simulink model "TPINVT"  (R2024b)
settings: Solver=VariableStepAuto  StartTime=0.0  StopTime=0.5  RelTol=1e-3
libraries: spsSeriesRLCBranchLib x6, spsVoltageMeasurementLib x3, spsCurrentMeasurementLib x2, spsDCVoltageSourceLib x1, simulink x1, spsUniversalBridgeLib x1, sps_lib x1
settings Model: Creator=李康诚  LastModifiedBy=86195
settings SolverCC: AlgebraicLoopSolver=TrustRegion
settings DebuggingCC: UnconnectedInputMsg=warning  UnconnectedOutputMsg=warning  UnconnectedLineMsg=warning
settings ModelReferenceCC: EnableRefExpFcnMdlSchedulingChecks=on
settings RTWCC: GPUComputeCapability=3.5  DLArmComputeVersion=19.05

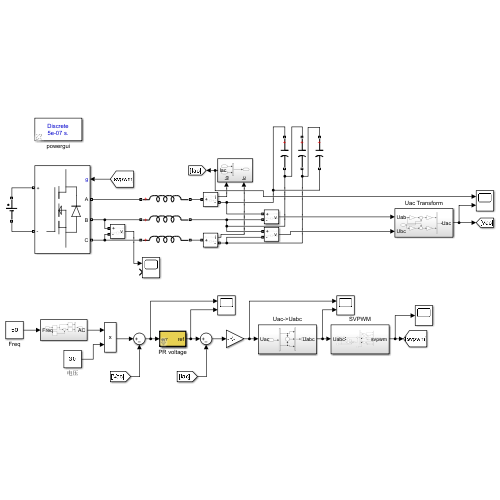
[thumbnail: Simulink's stored preview of the top-level diagram]
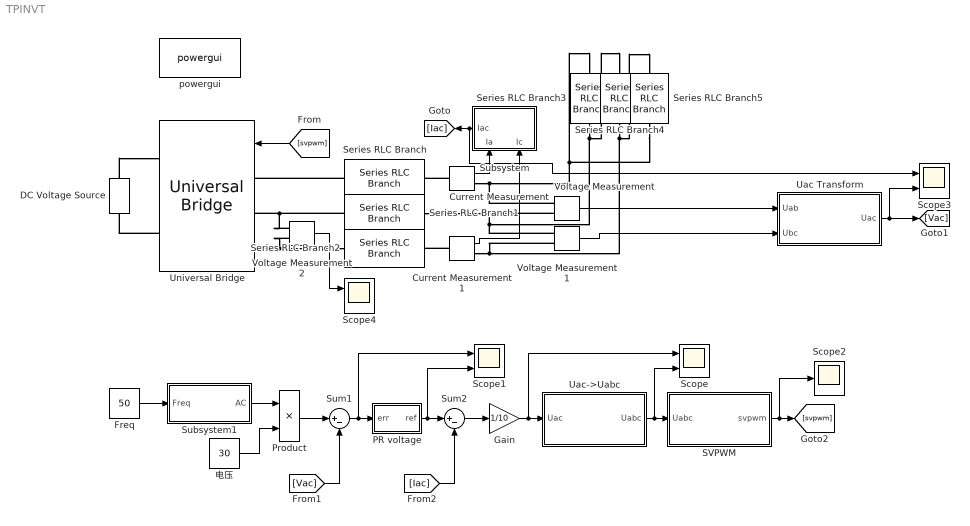
== system TPINVT ==
  Current Measurement : spsCurrentMeasurementLib/Current Measurement  PhasorSimulation=off  OutputType=Complex  PSBequivalent=0
  Current Measurement1 : spsCurrentMeasurementLib/Current Measurement  PhasorSimulation=off  OutputType=Complex  PSBequivalent=0
  DC Voltage Source : spsDCVoltageSourceLib/DC Voltage Source  Amplitude=50  Measurements=None
  Freq : Constant  Value=50
  Gain : Gain  Gain=1/10
  PR voltage : Subsystem  TreatAsAtomicUnit=on  mask{Kp=0.2, Kr=40, Wc=5, Upper=40, Lower=-40}
  Product : Product
  SVPWM : Subsystem
      settings: PortSchema="{\"entries\":[{\"content\":{\"sides\":[{\"content\":{\"connectorIds\":[\"Out1\"]},\"type\":\"ConnectorPlacement.EquallySpacedRectSide\",\"uuid\":\"dcbf9248-7910-4260-a5d4-f1c1a6bfbbe0\"},{\"content\":{\"connectorIds\":[\"In1\"],\"side\":\"RIGHT\"},\"type\":\"ConnectorPlacement.EquallySpacedRectSide\",\"uuid\":\"1c1c0724-ccc5-4c64-9077-43c2945212ef\"},{\"content\":{\"connectorIds\":[],\"side\":\"TOP\"},\"type\":\"ConnectorPlacement.EquallySpacedRectSide\",\"uuid\":\"9c7778fd-5bd1-45c2-a026-753aafe02b02\"},{\"content\":{\"connectorIds\":[],\"side\":\"HIDDEN\"},\"type\":\"ConnectorPlacement.EquallySpacedRectSide\",\"uuid\":\"bbcc7e5f-60a4-4189-91e6-d18a042c4fa5\"}]},\"type\":\"ConnectorPlacement.EquallySpacedConnector\",\"uuid\":\"5934fde8-9463-4fa5-a9de-717ebb1e8e0c\"}],\"packageUris\":[\"http://schema.mathworks.com/mf0/Connector/R2020b\"],\"version\":\"1.0\"}"
  Scope{,1,3..4} (4 alike) : Scope  NumInputPorts=2
  Scope2 : Scope
  Series RLC Branch : spsSeriesRLCBranchLib/Series RLC Branch  LConnTagsString=__new0  RConnTagsString=__new0  BranchType=L  Resistance=1  Inductance=1e-3  SetiL0=off  InitialCurrent=0  Capacitance=0  Setx0=off  InitialVoltage=0  Measurements=None
  Series RLC Branch1 : spsSeriesRLCBranchLib/Series RLC Branch  LConnTagsString=__new0  RConnTagsString=__new0  BranchType=L  Resistance=1  Inductance=1e-3  SetiL0=off  InitialCurrent=0  Capacitance=0  Setx0=off  InitialVoltage=0  Measurements=None
  Series RLC Branch2 : spsSeriesRLCBranchLib/Series RLC Branch  LConnTagsString=__new0  RConnTagsString=__new0  BranchType=L  Resistance=1  Inductance=1e-3  SetiL0=off  InitialCurrent=0  Capacitance=0  Setx0=off  InitialVoltage=0  Measurements=None
  Series RLC Branch3 : spsSeriesRLCBranchLib/Series RLC Branch  LConnTagsString=__new0  RConnTagsString=__new0  BranchType=C  Resistance=1  Inductance=1e-3  SetiL0=off  InitialCurrent=0  Capacitance=2e-6  Setx0=off  InitialVoltage=0  Measurements=None
  Series RLC Branch4 : spsSeriesRLCBranchLib/Series RLC Branch  LConnTagsString=__new0  RConnTagsString=__new0  BranchType=C  Resistance=1  Inductance=1e-3  SetiL0=off  InitialCurrent=0  Capacitance=2e-6  Setx0=off  InitialVoltage=0  Measurements=None
  Series RLC Branch5 : spsSeriesRLCBranchLib/Series RLC Branch  LConnTagsString=__new0  RConnTagsString=__new0  BranchType=C  Resistance=1  Inductance=1e-3  SetiL0=off  InitialCurrent=0  Capacitance=2e-6  Setx0=off  InitialVoltage=0  Measurements=None
  Subsystem : Subsystem
      settings: PortSchema="{\"entries\":[{\"content\":{\"sides\":[{\"content\":{\"connectorIds\":[\"In1\",\"In2\"]},\"type\":\"ConnectorPlacement.EquallySpacedRectSide\",\"uuid\":\"dcbf9248-7910-4260-a5d4-f1c1a6bfbbe0\"},{\"content\":{\"connectorIds\":[],\"side\":\"RIGHT\"},\"type\":\"ConnectorPlacement.EquallySpacedRectSide\",\"uuid\":\"1c1c0724-ccc5-4c64-9077-43c2945212ef\"},{\"content\":{\"connectorIds\":[\"Out1\"],\"side\":\"TOP\"},\"type\":\"ConnectorPlacement.EquallySpacedRectSide\",\"uuid\":\"9c7778fd-5bd1-45c2-a026-753aafe02b02\"},{\"content\":{\"connectorIds\":[],\"side\":\"HIDDEN\"},\"type\":\"ConnectorPlacement.EquallySpacedRectSide\",\"uuid\":\"bbcc7e5f-60a4-4189-91e6-d18a042c4fa5\"}]},\"type\":\"ConnectorPlacement.EquallySpacedConnector\",\"uuid\":\"5934fde8-9463-4fa5-a9de-717ebb1e8e0c\"}],\"packageUris\":[\"http://schema.mathworks.com/mf0/Connector/R2020b\"],\"version\":\"1.0\"}"
  Subsystem1 : Subsystem
  Sum1 : Sum  Inputs=|+-
  Sum2 : Sum  Inputs=|+-
  Uac Transform : Subsystem
      settings: PortSchema="{\"entries\":[{\"content\":{\"sides\":[{\"content\":{\"connectorIds\":[\"Out1\"]},\"type\":\"ConnectorPlacement.EquallySpacedRectSide\",\"uuid\":\"dcbf9248-7910-4260-a5d4-f1c1a6bfbbe0\"},{\"content\":{\"connectorIds\":[\"In1\",\"In2\"],\"side\":\"RIGHT\"},\"type\":\"ConnectorPlacement.EquallySpacedRectSide\",\"uuid\":\"1c1c0724-ccc5-4c64-9077-43c2945212ef\"},{\"content\":{\"connectorIds\":[],\"side\":\"TOP\"},\"type\":\"ConnectorPlacement.EquallySpacedRectSide\",\"uuid\":\"9c7778fd-5bd1-45c2-a026-753aafe02b02\"},{\"content\":{\"connectorIds\":[],\"side\":\"HIDDEN\"},\"type\":\"ConnectorPlacement.EquallySpacedRectSide\",\"uuid\":\"bbcc7e5f-60a4-4189-91e6-d18a042c4fa5\"}]},\"type\":\"ConnectorPlacement.EquallySpacedConnector\",\"uuid\":\"5934fde8-9463-4fa5-a9de-717ebb1e8e0c\"}],\"packageUris\":[\"http://schema.mathworks.com/mf0/Connector/R2020b\"],\"version\":\"1.0\"}"
  Uac->Uabc : Subsystem
      settings: PortSchema="{\"entries\":[{\"content\":{\"sides\":[{\"content\":{\"connectorIds\":[\"Out1\"]},\"type\":\"ConnectorPlacement.EquallySpacedRectSide\",\"uuid\":\"dcbf9248-7910-4260-a5d4-f1c1a6bfbbe0\"},{\"content\":{\"connectorIds\":[\"In1\"],\"side\":\"RIGHT\"},\"type\":\"ConnectorPlacement.EquallySpacedRectSide\",\"uuid\":\"1c1c0724-ccc5-4c64-9077-43c2945212ef\"},{\"content\":{\"connectorIds\":[],\"side\":\"TOP\"},\"type\":\"ConnectorPlacement.EquallySpacedRectSide\",\"uuid\":\"9c7778fd-5bd1-45c2-a026-753aafe02b02\"},{\"content\":{\"connectorIds\":[],\"side\":\"HIDDEN\"},\"type\":\"ConnectorPlacement.EquallySpacedRectSide\",\"uuid\":\"bbcc7e5f-60a4-4189-91e6-d18a042c4fa5\"}]},\"type\":\"ConnectorPlacement.EquallySpacedConnector\",\"uuid\":\"5934fde8-9463-4fa5-a9de-717ebb1e8e0c\"}],\"packageUris\":[\"http://schema.mathworks.com/mf0/Connector/R2020b\"],\"version\":\"1.0\"}"
  Universal Bridge : spsUniversalBridgeLib/Universal Bridge  Arms=3  SnubberResistance=1e5  SnubberCapacitance=inf  Device=MOSFET / Diodes  Ron=0.01  Lon=0  ForwardVoltages="[  0  0  ]"  ForwardVoltage=0  GTOparameters=[ 10e-6 , 20e-6 ]  IGBTparameters=[ 1e-6 , 2e-6 ]  Measurements=None  Measurements_2=None  converterType=Rectifier
  Voltage Measurement : spsVoltageMeasurementLib/Voltage Measurement  PhasorSimulation=off  OutputType=Complex  PSBequivalent=0
  Voltage Measurement1 : spsVoltageMeasurementLib/Voltage Measurement  PhasorSimulation=off  OutputType=Complex  PSBequivalent=0
  Voltage Measurement2 : spsVoltageMeasurementLib/Voltage Measurement  PhasorSimulation=off  OutputType=Complex  PSBequivalent=0
  powergui : sps_lib/powergui  Priority=1  SimulationMode=Discrete  SampleTime=5e-7  frequency=60  Iterations=50  frequencyindice=0  Pbase=100e6  ErrMax=1e-4  UnitsV=kV  UnitsW=MW  buscounter=0  FunctionMessages=off  echomessages=off  EnableUseOfTLC=off  CurrentSourceSwitches=off  DisableSnubberDevices=off  DisableRonSwitches=off  DisableVfSwitches=off  DisplayEquations=off  AutomaticDiscreteSolvers=off  SolverType=Tustin/Backward Euler (TBE)  Interpol=off  ExternalGateDelay=off  methode=off  Ts=100  x0status=blocks  SPID=on  SwTol=0  HookPort=off  NonlinearTolerance=1e-4  nMaxIteration=100  ContinueOnMaxIteration=off  RestoreLinks=warning  ResistiveCurrentMeasurement=off  Frange=[0:2:500]  Ylog=off  Xlog=on  ShowGrid=off  save=off  variable=ZData  structure=0  ZoomFFT=off  StartTime=0.0  cycles=1  DisplayStyle=1  fundamental=60  FreqAxis=off  MaxFrequency=1000  frequencyindicesteady=1  RmsSteady=1  display=off
  电压 : Constant  Value=30
  wires:
  [svpwm] -> Universal Bridge/1
  Current Measurement/1 -> Subsystem/1(Ia)
  Current Measurement1/1 -> Subsystem/2(Ic)
  Subsystem/1(Iac) -> Scope3/1, [Iac]
  Freq/1 -> Subsystem1/1(Freq)
  Subsystem1/1(AC) -> Product/1
  电压/1 -> Product/2
  Product/1 -> Sum1/1
  [Vac] -> Sum1/2
  [Iac] -> Sum2/2
  Sum2/1 -> Gain/1
  Uac Transform/1(Uac) -> [Vac], Scope3/2
  Voltage Measurement/1 -> Uac Transform/1(Uab)
  Voltage Measurement1/1 -> Uac Transform/2(Ubc)
  Gain/1 -> Scope/1, Uac->Uabc/1(Uac)
  Uac->Uabc/1(Uabc) -> Scope/2, SVPWM/1(Uabc)
  SVPWM/1(svpwm) -> Scope2/1, [svpwm]
  Sum1/1 -> Scope1/1, PR voltage/1(err)
  PR voltage/1(ref) -> Scope1/2, Sum2/1
  Voltage Measurement2/1 -> Scope4/1
  connections:
  DC Voltage Source/RConn1 -- Universal Bridge/RConn1
  Universal Bridge/RConn2 -- DC Voltage Source/LConn1
  Series RLC Branch/LConn1 -- Universal Bridge/LConn1
  Series RLC Branch1/LConn1 -- Voltage Measurement2/LConn1 -- Universal Bridge/LConn2
  Current Measurement/LConn1 -- Series RLC Branch/RConn1
  Current Measurement/RConn1 -- Voltage Measurement/LConn1 -- Series RLC Branch3/LConn1 -- Series RLC Branch5/RConn1
  Current Measurement1/LConn1 -- Series RLC Branch2/RConn1
  Series RLC Branch3/RConn1 -- Voltage Measurement1/LConn1 -- Series RLC Branch1/RConn1 -- Voltage Measurement/LConn2 -- Series RLC Branch4/LConn1
  Series RLC Branch4/RConn1 -- Voltage Measurement1/LConn2 -- Current Measurement1/RConn1 -- Series RLC Branch5/LConn1
  Universal Bridge/LConn3 -- Voltage Measurement2/LConn2 -- Series RLC Branch2/LConn1

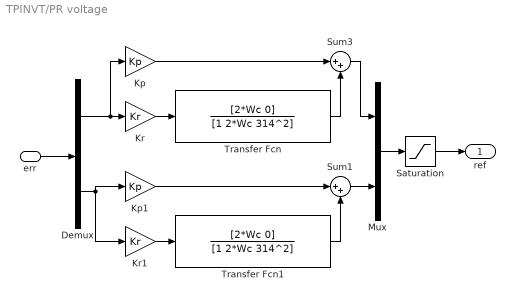
== system TPINVT/PR voltage ==
  err : Inport
  Demux : Demux  Outputs=2
  Kp : Gain  Gain=Kp
  Kp1 : Gain  Gain=Kp
  Kr : Gain  Gain=Kr
  Kr1 : Gain  Gain=Kr
  Mux : Mux  Inputs=2
  Saturation : Saturate  UpperLimit=Upper  LowerLimit=Lower
  Sum1 : Sum  Inputs=|++
  Sum3 : Sum  Inputs=|++
  Transfer Fcn : TransferFcn  Numerator=[2*Wc 0]  Denominator=[1 2*Wc 314^2]
  Transfer Fcn1 : TransferFcn  Numerator=[2*Wc 0]  Denominator=[1 2*Wc 314^2]
  ref : Outport
  wires:
  Kp/1 -> Sum3/1
  Kr/1 -> Transfer Fcn/1
  Transfer Fcn/1 -> Sum3/2
  Saturation/1 -> ref/1
  err/1 -> Demux/1
  Demux/1 -> Kr/1, Kp/1
  Sum3/1 -> Mux/1
  Mux/1 -> Saturation/1
  Demux/2 -> Kr1/1, Kp1/1
  Transfer Fcn1/1 -> Sum1/2
  Kr1/1 -> Transfer Fcn1/1
  Kp1/1 -> Sum1/1
  Sum1/1 -> Mux/2

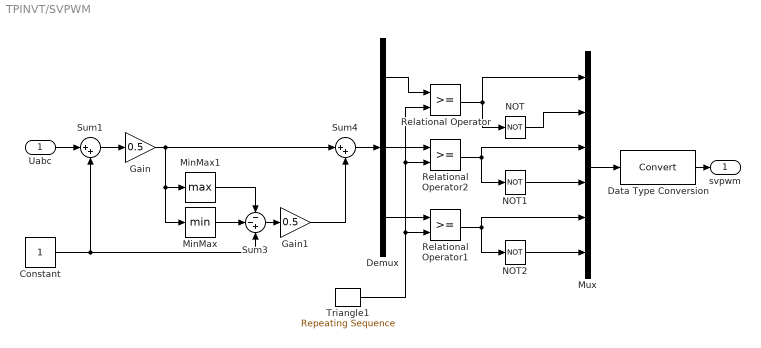
== system TPINVT/SVPWM ==
  Uabc : Inport
  Constant : Constant
  Data Type Conversion : DataTypeConversion  SaturateOnIntegerOverflow=off  RndMeth=Floor
  Demux : Demux  Outputs=3
  Gain : Gain  Gain=0.5
  Gain1 : Gain  Gain=0.5
  MinMax : MinMax
  MinMax1 : MinMax  Function=max
  Mux : Mux  Inputs=6
  NOT : Logic  Operator=NOT  IconShape=distinctive  AllPortsSameDT=off  OutDataTypeStr=boolean
  NOT1 : Logic  Operator=NOT  IconShape=distinctive  AllPortsSameDT=off  OutDataTypeStr=boolean
  NOT2 : Logic  Operator=NOT  IconShape=distinctive  AllPortsSameDT=off  OutDataTypeStr=boolean
  Relational Operator : RelationalOperator  OutDataTypeStr=boolean  InputSameDT=off
  Relational Operator1 : RelationalOperator  OutDataTypeStr=boolean  InputSameDT=off
  Relational Operator2 : RelationalOperator  OutDataTypeStr=boolean  InputSameDT=off
  Sum1 : Sum  Inputs=|++
  Sum3 : Sum  Inputs=--+
  Sum4 : Sum  Inputs=|++
  Triangle1 : simulink/Sources/Repeating Sequence  rep_seq_t=[0 1/16000/2 1/16000]  rep_seq_y=[0 2 0]
  svpwm : Outport
  wires:
  Uabc/1 -> Sum1/1
  Sum1/1 -> Gain/1
  Constant/1 -> Sum3/3, Sum1/2
  Gain/1 -> Sum4/1, MinMax/1, MinMax1/1
  MinMax1/1 -> Sum3/1
  MinMax/1 -> Sum3/2
  Sum3/1 -> Gain1/1
  Gain1/1 -> Sum4/2
  Sum4/1 -> Demux/1
  NOT1/1 -> Mux/4
  Relational Operator2/1 -> NOT1/1, Mux/3
  NOT/1 -> Mux/2
  Demux/2 -> Relational Operator2/1
  Relational Operator/1 -> NOT/1, Mux/1
  Demux/1 -> Relational Operator/1
  NOT2/1 -> Mux/6
  Relational Operator1/1 -> Mux/5, NOT2/1
  Demux/3 -> Relational Operator1/1
  Triangle1/1 -> Relational Operator1/2, Relational Operator2/2, Relational Operator/2
  Mux/1 -> Data Type Conversion/1
  Data Type Conversion/1 -> svpwm/1

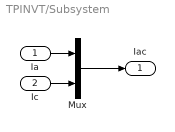
== system TPINVT/Subsystem ==
  Ia : Inport
  Ic : Inport  Port=2
  Mux : Mux  Inputs=2
  Iac : Outport
  wires:
  Mux/1 -> Iac/1
  Ic/1 -> Mux/2
  Ia/1 -> Mux/1

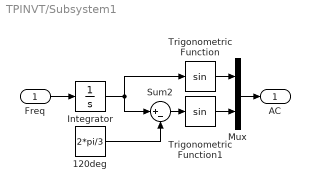
== system TPINVT/Subsystem1 ==
  Freq : Inport
  120deg : Constant  Value=2*pi/3
  Integrator : Integrator  WrapState=on  WrappedStateUpperValue=2*pi  WrappedStateLowerValue=0
  Mux : Mux  Inputs=2
  Sum2 : Sum  Inputs=|+-
  Trigonometric Function : Trigonometry
  Trigonometric Function1 : Trigonometry
  AC : Outport
  wires:
  Integrator/1 -> Trigonometric Function/1, Sum2/1
  Trigonometric Function/1 -> Mux/1
  Sum2/1 -> Trigonometric Function1/1
  120deg/1 -> Sum2/2
  Trigonometric Function1/1 -> Mux/2
  Mux/1 -> AC/1
  Freq/1 -> Integrator/1

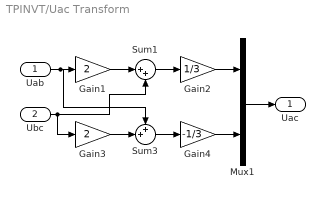
== system TPINVT/Uac Transform ==
  Uab : Inport
  Ubc : Inport  Port=2
  Gain1 : Gain  Gain=2
  Gain2 : Gain  Gain=1/3
  Gain3 : Gain  Gain=2
  Gain4 : Gain  Gain=-1/3
  Mux1 : Mux  Inputs=2
  Sum1 : Sum  Inputs=|++
  Sum3 : Sum  Inputs=++|
  Uac : Outport
  wires:
  Gain1/1 -> Sum1/1
  Sum1/1 -> Gain2/1
  Gain2/1 -> Mux1/1
  Mux1/1 -> Uac/1
  Uab/1 -> Sum3/1, Gain1/1
  Ubc/1 -> Gain3/1, Sum1/2
  Sum3/1 -> Gain4/1
  Gain3/1 -> Sum3/2
  Gain4/1 -> Mux1/2

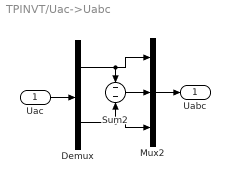
== system TPINVT/Uac->Uabc ==
  Uac : Inport
  Demux : Demux  Outputs=2
  Mux2 : Mux  Inputs=3
  Sum2 : Sum  Inputs=-|-
  Uabc : Outport
  wires:
  Uac/1 -> Demux/1
  Demux/1 -> Mux2/1, Sum2/1
  Demux/2 -> Sum2/2, Mux2/3
  Sum2/1 -> Mux2/2
  Mux2/1 -> Uabc/1
